simulink model "PID_aircraft_pitch_control"  (R2020b)
settings: Solver=VariableStepAuto  StartTime=0.0  StopTime=25  RelTol=1e-3
undefined symbols (not defined in the file): Earth, WGS84
libraries: aerolibfltsims x2, pid_lib x1, aerolibtransform2 x1
settings Model: Creator=GURU  LastModifiedBy=GURU

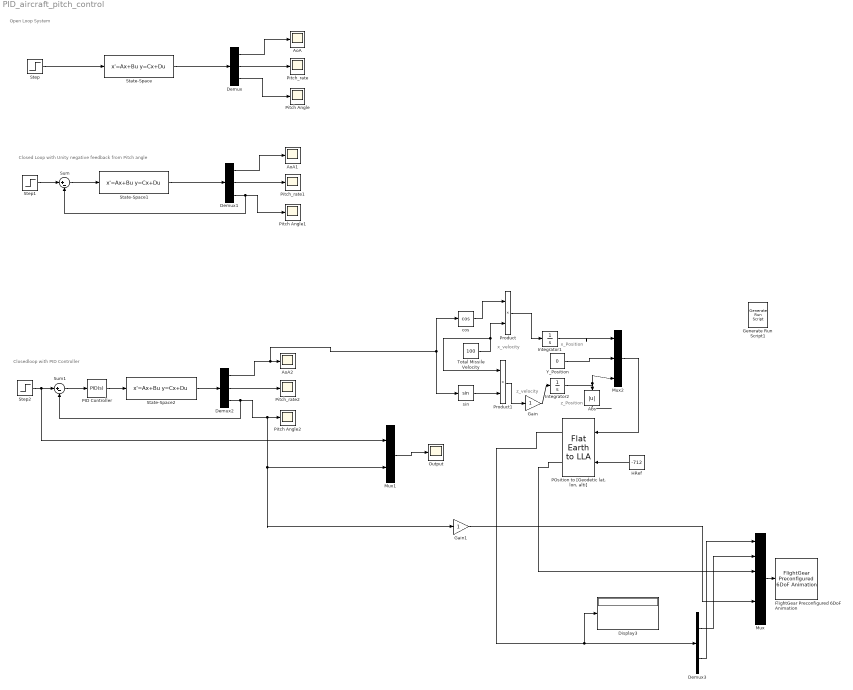
== system PID_aircraft_pitch_control ==
  note: Closedloop with PID Controller
  note: Closed Loop with Unity negative feedback from Pitch angle
  note: Open Loop System
  note: z_Position
  note: z_velocity
  note: x_velocity
  note: x_Position
  Abs : Abs
  AoA : Scope
  AoA1 : Scope
  AoA2 : Scope
  Demux : Demux  Outputs=3
  Demux1 : Demux  Outputs=3
  Demux2 : Demux  Outputs=3
  Demux3 : Demux  Outputs=2
  Display3 : Display
      settings: Decimation=2
  FlightGear Preconfigured 6DoF Animation : aerolibfltsims/FlightGear Preconfigured 6DoF Animation  xFlightGearVersion=v2019.1  DestinationIpAddress=127.0.0.1  DestinationPort=5502  SampleTime=1/30  packetVersion=24
  Gain : Gain
  Gain1 : Gain
  Generate Run Script1 : aerolibfltsims/Generate Run Script  Architecture=Win64  dataFlow=Send  GeometryModelName=c172p  AirportId=KSFO  RunwayId=10L  InitialAltitude=7224  InitialHeading=113  OffsetDistance=4.72  OffsetAzimuth=0  InstallScenery=on  DisableShaders=on  OriginAddress=127.0.0.1  DestinationPort=5502  OriginPort=5505  LocalAddress=127.0.0.1  OutputFileName=runfg.bat  FlightGearBaseDirectory=C:\Program Files\FlightGear
  HRef : Constant  Value=-712
  Integrator1 : Integrator
  Integrator2 : Integrator  InitialCondition=-500
  Mux : Mux  Inputs=6
  Mux1 : Mux  Inputs=2
  Mux2 : Mux  Inputs=3
  Output : Scope
  PID Controller : pid_lib/PID Controller  Controller=PID  Form=Parallel  TimeDomain=Continuous-time  UseExternalTs=off  SampleTime=-1  IntegratorMethod=Forward Euler  FilterMethod=Forward Euler  ControllerParametersSource=internal  P=1.41625946995747  I=0.220101565523826  D=2.2200684913915  UseFilter=on  N=321.97973743592  TunerSelectOption=Transfer Function Based (PID Tuner App)  InitialConditionSource=internal  InitialConditionForIntegrator=0  InitialConditionForFilter=0  DifferentiatorICPrevScaledInput=0  ExternalReset=none  TrackingMode=off  Kt=1  LimitOutput=on  SatLimitsSource=internal  UpperSaturationLimit=0.4363  LowerSaturationLimit=-.4363  LinearizeAsGain=on  AntiWindupMode=none  Kb=1  POutMin=[]  POutMax=[]  IOutMin=[]  IOutMax=[]  DOutMin=[]  DOutMax=[]  NOutMin=[]  NOutMax=[]  SumOutMin=[]  SumOutMax=[]  SaturationOutMin=[]  SaturationOutMax=[]  PParamMin=[]  PParamMax=[]  IParamMin=[]  IParamMax=[]  DParamMin=[]  DParamMax=[]  NParamMin=[]  NParamMax=[]  KbParamMin=[]  KbParamMax=[]  KtParamMin=[]  KtParamMax=[]  KbOutMin=[]  KbOutMax=[]  KtOutMin=[]  KtOutMax=[]  IntegratorOutMin=[]  IntegratorOutMax=[]  FilterOutMin=[]  FilterOutMax=[]  SumI1OutMin=[]  SumI1OutMax=[]  SumI2OutMin=[]  SumI2OutMax=[]  SumI3OutMin=[]  SumI3OutMax=[]  SumI4OutMin=[]  SumI4OutMax=[]  SumDOutMin=[]  SumDOutMax=[]  DifferentiatorOutMin=[]  DifferentiatorOutMax=[]  FilterDiffOutCoefMin=[]  FilterDiffOutCoefMax=[]  ReciprocalOutMin=[]  ReciprocalOutMax=[]  SumDenOutMin=[]  SumDenOutMax=[]  SumNumOutMin=[]  SumNumOutMax=[]  DivideOutMin=[]  DivideOutMax=[]  UdiffTsProdOutMin=[]  UdiffTsProdOutMax=[]  NTsProdOutMin=[]  NTsProdOutMax=[]  UintegralTsProdOutMin=[]  UintegralTsProdOutMax=[]  UngainTsProdOutMin=[]  UngainTsProdOutMax=[]  IntegratorContinuousStateAttributes=''  IntegratorStateMustResolveToSignalObject=off  IntegratorRTWStateStorageClass=Auto  FilterContinuousStateAttributes=''  FilterStateMustResolveToSignalObject=off  FilterRTWStateStorageClass=Auto  ParallelPVariant=InternalParameters  IdealPVariant=Disabled  IVariant=InternalParameters  DVariant=InternalParameters  IntegratorVariant=Continuous  SatVariant=Enabled  AWVariant=Passthrough  PCopyVariant=Disabled  TRVariant=Disabled  FdbkBlocksVariant=Forward  IdealPFdbkVariant=Disabled  SatFdbkVariant=Disabled  DerivativeFilterVariant=ContFilter  NVariant=InternalParameters  NCopyVariant=Disabled  FilterICVariant=InternalICsFilter  IntegratorICVariant=InternalICs  ExternalResetVariant=Disabled  TRSumVariant=Passthrough  SumFdbkVariant=Disabled  SumVariant=Sum_PID  TsampFilterVariant=InternalTs  TsampNgainVariant=Passthrough  TsampIntegralVariant=Passthrough  ExternalSaturationOutDataTypeStr=Inherit: Same as second input
  "POsition to [Geodetic lat, lon, alti]" : aerolibtransform2/Flat Earth to LLA  units=Metric (MKS)  ptype=Earth (WGS84)  F=1/298.257223563  R=6378137  refPosPort=off  LL0=[34.910 -117.8912]  psi=0
  Pitch Angle : Scope
  Pitch Angle1 : Scope
  Pitch Angle2 : Scope
  Pitch_rate : Scope
  Pitch_rate1 : Scope
  Pitch_rate2 : Scope
  Product : Product
  Product1 : Product
  State-Space : StateSpace  A=[-0.313 56.7 0; -0.0139 -0.426 0; 0 56.7 0]  B=[0.232; 0.0203; 0]  C=eye(3)  D=[0;0;0]  InitialCondition=0  ContinuousStateAttributes={'aoa', 'pitch_rate', 'pitch_angle'}
  State-Space1 : StateSpace  A=[-0.313 56.7 0; -0.0139 -0.426 0; 0 56.7 0]  B=[0.232; 0.0203; 0]  C=eye(3)  D=[0;0;0]  InitialCondition=0  ContinuousStateAttributes={'aoa', 'pitch_rate', 'pitch_angle'}
  State-Space2 : StateSpace  A=[-0.313 56.7 0; -0.0139 -0.426 0; 0 56.7 0]  B=[0.232; 0.0203; 0]  C=eye(3)  D=[0;0;0]  InitialCondition=0  ContinuousStateAttributes={'aoa', 'pitch_rate', 'pitch_angle'}
  Step : Step  Time=0  SampleTime=0
  Step1 : Step  Time=0  SampleTime=0
  Step2 : Step  Time=0  After=0.25  SampleTime=0
  Sum : Sum  Inputs=|+-
  Sum1 : Sum  Inputs=|+-
  Total Missile Velocity : Constant  Value=100
  Y_Position : Constant  Value=0
  cos : Trigonometry  Operator=cos
  sin : Trigonometry
  wires:
  Step/1 -> State-Space/1
  State-Space/1 -> Demux/1
  Demux/1 -> AoA/1
  Demux/2 -> Pitch_rate/1
  Demux/3 -> Pitch Angle/1
  Demux1/3 -> Pitch Angle1/1, Sum/2
  Demux1/2 -> Pitch_rate1/1
  Demux1/1 -> AoA1/1
  State-Space1/1 -> Demux1/1
  Step1/1 -> Sum/1
  Sum/1 -> State-Space1/1
  Sum1/1 -> PID Controller/1
  Step2/1 -> Mux1/1, Sum1/1
  PID Controller/1 -> State-Space2/1
  State-Space2/1 -> Demux2/1
  Demux2/3 -> Sum1/2, Mux1/2, Gain1/1, Pitch Angle2/1
  Demux2/2 -> Pitch_rate2/1
  Integrator2/1 -> Mux2/3, Abs/1
  "POsition to [Geodetic lat, lon, alti]"/1 -> Display3/1, Demux3/1
  Demux2/1 -> sin/1, cos/1, AoA2/1
  "POsition to [Geodetic lat, lon, alti]"/2 -> Mux/3
  Abs/1 -> ?
  Demux3/2 -> Mux/1
  cos/1 -> Product/1
  Gain/1 -> Integrator2/1
  Mux2/1 -> "POsition to [Geodetic lat, lon, alti]"/1
  Demux3/1 -> Mux/2
  Mux/1 -> FlightGear Preconfigured 6DoF Animation/1
  Integrator1/1 -> Mux2/1
  Y_Position/1 -> Mux2/2
  sin/1 -> Product1/2
  HRef/1 -> "POsition to [Geodetic lat, lon, alti]"/2
  Total Missile Velocity/1 -> Product1/1, Product/2
  Product/1 -> Integrator1/1
  Product1/1 -> Gain/1
  Mux1/1 -> Output/1
  Gain1/1 -> Mux/5
